simulink model "RLC_Sim"  (R2022b)
settings: Solver=VariableStepAuto  StartTime=0.0  StopTime=10  RelTol=1e-3
values from neighbouring files (symbols this model uses):
  C = 1    [RLC_Parameters.m]
  L = 1    [RLC_Parameters.m]
  R = 2    [RLC_Parameters.m]
  v = 5    [RLC_Parameters.m]
settings Model: Creator=Sergio  LastModifiedBy=c.hernandez
settings SolverCC: AlgebraicLoopSolver=TrustRegion
settings DataIOCC: ReturnWorkspaceOutputs=off
settings DebuggingCC: UnconnectedInputMsg=warning  UnconnectedOutputMsg=warning  UnconnectedLineMsg=warning  SFMachineParentedDataDiag=warning  ArithmeticOperatorsInVariantConditions=warning
settings ModelReferenceCC: EnableRefExpFcnMdlSchedulingChecks=on
settings SFSimCC: SimUseLocalCustomCode=off  CustomCodeUndefinedFunction=UseInterfaceOnly
settings RTWCC: RTWUseLocalCustomCode=off  DLArmComputeVersion=19.05

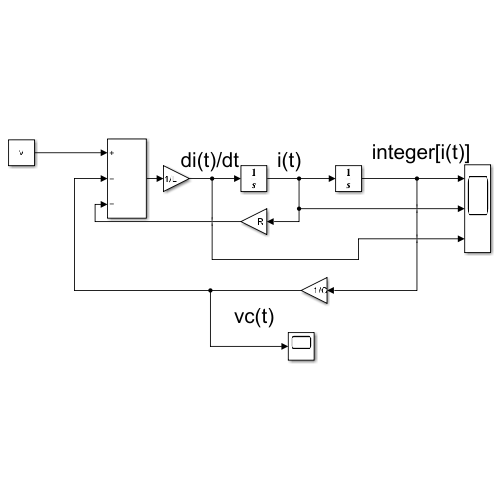
[thumbnail: Simulink's stored preview of the top-level diagram]
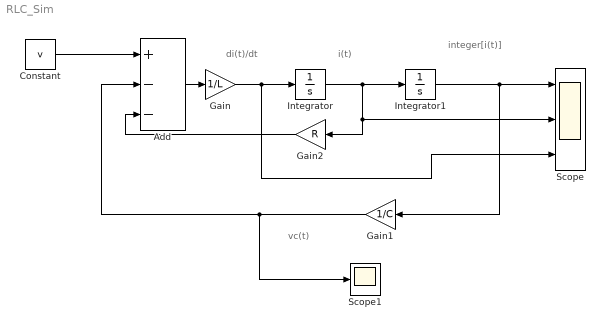
== system RLC_Sim ==
  note: di(t)/dt
  note: i(t)
  note: integer[i(t)]
  note: vc(t)
  Add : Sum  Inputs=+--
  Constant : Constant  Value=v
  Gain : Gain  Gain=1/L
  Gain1 : Gain  Gain=1/C
  Gain2 : Gain  Gain=R
  Integrator : Integrator
  Integrator1 : Integrator
  Scope : Scope  NumInputPorts=3
  Scope1 : Scope
  wires:
  Gain/1 -> Scope/3, Integrator/1
  Integrator/1 -> Integrator1/1, Gain2/1, Scope/2
  Integrator1/1 -> Gain1/1, Scope/1
  Constant/1 -> Add/1
  Gain2/1 -> Add/3
  Gain1/1 -> Scope1/1, Add/2
  Add/1 -> Gain/1
